simulink model "EinwegGleichrichter_"  (Simulink 8.4)
settings: Solver=ode4  StartTime=0.0  StopTime=10  FixedStep=1e-3  MaxStep=1e-4  RelTol=1e-3
libraries: dsparch4 x3
settings Model: Creator=Administrator  LastModifiedBy=Administrator
settings DataIOCC: SignalLoggingName=sigsOut
settings OptimizationCC: ExpressionDepthLimit=128
settings DebuggingCC: SaveWithParameterizedLinksMsg=none  SignalResolutionControl=TryResolveAllWithWarning  SolverPrmCheckMsg=none  MultiTaskDSMMsg=warning  MultiTaskCondExecSysMsg=none  FcnCallInpInsideContextMsg=EnableAllAsError  StateNameClashWarn=none
settings HardwareCC: TargetUnknown=on
settings RTWCC: IncludeERTFirstTime=on

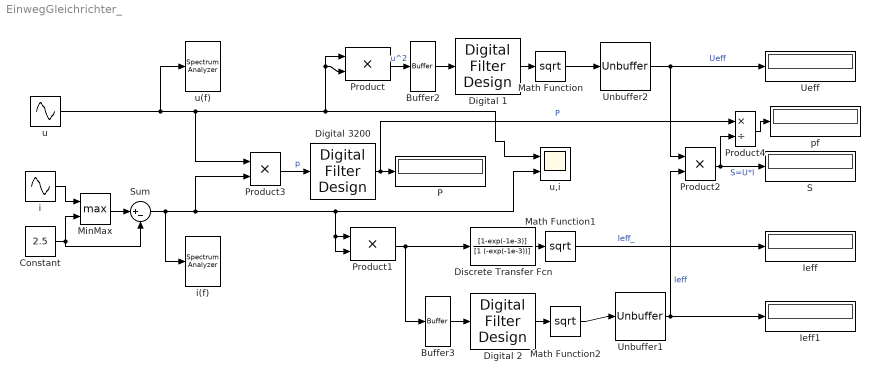
== system EinwegGleichrichter_ ==
  Buffer2 : Buffer  N=256
  Buffer3 : Buffer  N=256
  Constant : Constant  Value=2.5
  Digital 1 : dsparch4/Digital Filter Design  mwdsp_browser_bugfix_var=off
  Digital 2 : dsparch4/Digital Filter Design  mwdsp_browser_bugfix_var=off
  Digital 3200 : dsparch4/Digital Filter Design  mwdsp_browser_bugfix_var=off
  Discrete Transfer Fcn : DiscreteTransferFcn  Numerator=[1-exp(-1e-3)]  Denominator=[1 (-exp(-1e-3))]
  Ieff : Display
  Ieff1 : Display
  Math Function : Math  Operator=sqrt  SaturateOnIntegerOverflow=on
  Math Function1 : Math  Operator=sqrt  SaturateOnIntegerOverflow=on
  Math Function2 : Math  Operator=sqrt  SaturateOnIntegerOverflow=on
  MinMax : MinMax  Function=max  Inputs=2  SaturateOnIntegerOverflow=on  InputSameDT=on
  P : Display
  Product{,1..3} (4 alike) : Product  SaturateOnIntegerOverflow=on  OutDataTypeStr=Inherit: Same as first input
  Product4 : Product  Inputs=*/  SaturateOnIntegerOverflow=on  OutDataTypeStr=Inherit: Same as first input
  S : Display
  Sum : Sum  Inputs=|+-  SaturateOnIntegerOverflow=on
  Ueff : Display
  Unbuffer1 : Unbuffer
  Unbuffer2 : Unbuffer
  i : Sin  SineType=Sample based  Amplitude=311/100  Frequency=314  Samples=20  SampleTime=1e-3
  i(f) : SpectrumAnalyzer
  pf : Display
  u : Sin  SineType=Sample based  Amplitude=230*2^0.5  Frequency=314  Samples=20  SampleTime=1e-3
  u(f) : SpectrumAnalyzer
  u,i : Scope  NumInputPorts=2
      settings: YMin=-5~-5  YMax=5~5
  wires:
  i/1 -> MinMax/1
  Constant/1 -> MinMax/2, Sum/2
  Product/1 -> Buffer2/1  "u^2"
  Digital 1/1 -> Math Function/1
  Product1/1 -> Discrete Transfer Fcn/1, Buffer3/1
  Discrete Transfer Fcn/1 -> Math Function1/1
  Product3/1 -> Digital 3200/1  "p"
  Digital 3200/1 -> P/1, Product4/1  "P"
  Math Function/1 -> Unbuffer2/1
  Math Function1/1 -> Ieff/1  "Ieff_"
  u/1 -> Product3/1, Product/2, Product/1, u,i/1, u(f)/1
  Buffer2/1 -> Digital 1/1
  Digital 2/1 -> Math Function2/1
  Buffer3/1 -> Digital 2/1
  Math Function2/1 -> Unbuffer1/1
  Unbuffer1/1 -> Ieff1/1, Product2/2  "Ieff"
  Unbuffer2/1 -> Ueff/1, Product2/1  "Ueff"
  Product2/1 -> S/1, Product4/2  "S=U*I"
  Product4/1 -> pf/1
  MinMax/1 -> Sum/1
  Sum/1 -> i(f)/1, Product3/2, u,i/2, Product1/1, Product1/2
